simulink model "lab1_2"  (R2021a)
settings: Solver=VariableStepAuto  StartTime=0.0  StopTime=100.0  RelTol=1e-10  AbsTol=1e-10
values from neighbouring files (symbols this model uses):
  den1 = cell2mat(den1)    [lab1.m]
  num1 = cell2mat(num1)    [lab1.m]
settings Model: Creator=markalex  LastModifiedBy=markalex

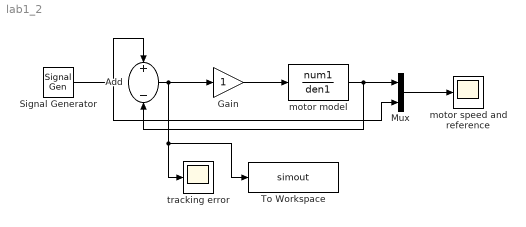
== system lab1_2 ==
  Add : Sum  Inputs=+-
  Gain : Gain
  Mux : Mux  Inputs=2
  Signal Generator : SignalGenerator  WaveForm=square  Frequency=0.02
  To Workspace : ToWorkspace  VariableName=simout  SaveFormat=Timeseries  SampleTime=-1
  motor model : TransferFcn  Numerator=num1  Denominator=den1
  motor speed and reference : Scope
  tracking error : Scope
  wires:
  Signal Generator/1 -> Add/1, Mux/2
  Add/1 -> tracking error/1, To Workspace/1, Gain/1
  Gain/1 -> motor model/1
  motor model/1 -> Add/2, Mux/1
  Mux/1 -> motor speed and reference/1
